simulink model "TGFF_checkout"  (Simulink 9.2)
settings: Solver=FixedStepDiscrete  StartTime=0.0  StopTime=10  FixedStep=SIM_dt  RelTol=1e-3
values from neighbouring files (symbols this model uses):
  SIM_dt = 0.01    [init_secOrdFilt_checkout.m]    (also in init_secOrdSS_checkout.m = 0.001)
undefined symbols (not defined in the file or in its folder): TGFF_B, TGFF_CmdLim_lb, TGFF_CmdLim_ub, TGFF_Coul_Nm, TGFF_Gain, TGFF_J, TGFF_K, TGFF_Kf, TGFF_MomArm, TGFF_Visc_Nmsprad
libraries: simulink x1
settings Model: Creator=coewal  LastModifiedBy=coewal
settings DataIOCC: LimitDataPoints=off  SaveFormat=Dataset  SignalLoggingSaveFormat=Dataset
settings OptimizationCC: LifeSpan=auto
settings DebuggingCC: UnderspecifiedInitializationDetection=Simplified  MergeDetectMultiDrivingBlocksExec=error  FcnCallInpInsideContextMsg=error  StateNameClashWarn=none  SFUnexpectedBacktrackingDiag=error  SFNoUnconditionalDefaultTransitionDiag=error  SFExecutionAtInitializationDiag=warning
settings HardwareCC: ProdBitPerPointer=64  ProdBitPerSizeT=64  ProdBitPerPtrDiffT=64  ProdLargestAtomicFloat=Float  ProdIntDivRoundTo=Zero  ProdEndianess=LittleEndian  ProdWordSize=64  ProdHWDeviceType=Intel->x86-64 (Windows64)
settings ModelReferenceCC: PropagateSignalLabelsOutOfModel=on
settings SFSimCC: SimUseLocalCustomCode=on
settings RTWCC: RTWUseLocalCustomCode=on
settings CodeAppCC: StateflowObjectComments=off
settings GRTTargetCC: TargetLangStandard=C99 (ISO)  GeneratePreprocessorConditionals=Use local settings  CombineOutputUpdateFcns=on  GRTInterface=off
settings ConfigComp: CovMetricSettings=dwe  CovHtmlReporting=off  CovSaveCumulativeToWorkspaceVar=off  CovSaveSingleToWorkspaceVar=off  CovExternalEMLEnable=on

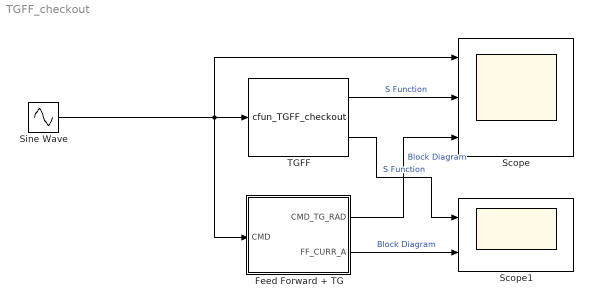
== system TGFF_checkout ==
  Feed Forward + TG : Subsystem
  Scope : Scope  NumInputPorts=3
  Scope1 : Scope  NumInputPorts=2
  Sine Wave : Sin  Amplitude=pi/180  Frequency=5  SampleTime=SIM_dt
  TGFF : S-Function  FunctionName=cfun_TGFF_checkout  Parameters=SIM_dt,TGFF_K,TGFF_B,TGFF_J,TGFF_MomArm,TGFF_Kf,TGFF_Gain,TGFF_CmdLim_ub,TGFF_CmdLim_lb,TGFF_Coul_Nm,TGFF_Visc_Nmsprad  SFunctionModules='TGFF'  SFunctionDeploymentMode=off  EnableBusSupport=off
  wires:
  TGFF/1 -> Scope/2  "S Function"
  Sine Wave/1 -> Feed Forward + TG/1(CMD), Scope/1, TGFF/1
  Feed Forward + TG/2(FF_CURR_A) -> Scope1/2  "Block Diagram"
  Feed Forward + TG/1(CMD_TG_RAD) -> Scope/3  "Block Diagram"
  TGFF/2 -> Scope1/1  "S Function"

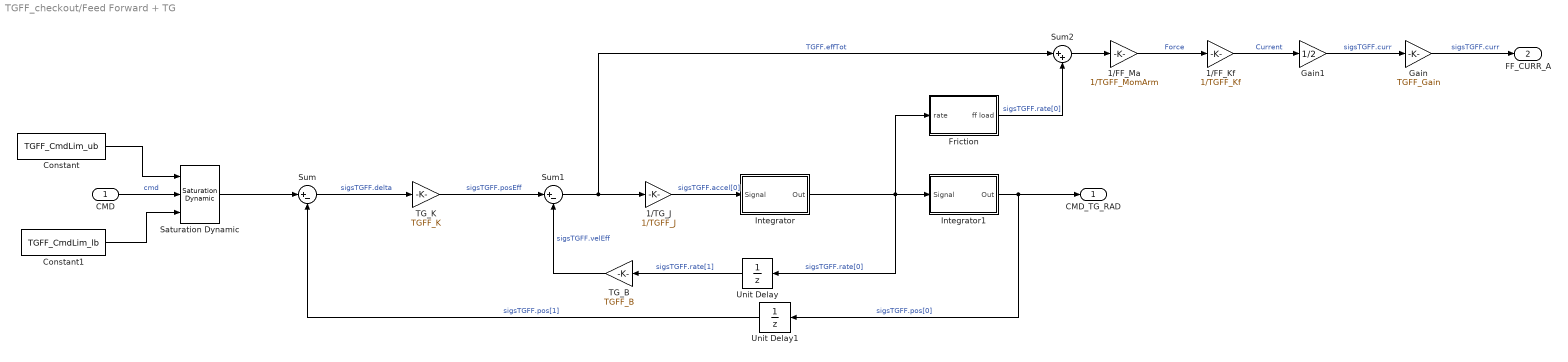
== system TGFF_checkout/Feed Forward + TG ==
  CMD : Inport
  1/FF_Kf : Gain  Gain=1/TGFF_Kf
  1/FF_Ma : Gain  Gain=1/TGFF_MomArm
  1/TG_J : Gain  Gain=1/TGFF_J
  Constant : Constant  Value=TGFF_CmdLim_ub  SampleTime=SIM_dt
  Constant1 : Constant  Value=TGFF_CmdLim_lb  SampleTime=SIM_dt
  Friction : Subsystem
  Gain : Gain  Gain=TGFF_Gain
  Gain1 : Gain  Gain=1/2
  Integrator : Subsystem
  Integrator1 : Subsystem
  Saturation Dynamic : simulink/Discontinuities/Saturation Dynamic  OutMin=[]  OutMax=[]  OutDataTypeStr=Inherit: Same as second input  OutDataType=fixdt(1, 16)  OutScaling=2^-10  DoSatur=off
  Sum : Sum  Inputs=|+-
  Sum1 : Sum  Inputs=|+-
  Sum2 : Sum  Inputs=|++
  TG_B : Gain  Gain=TGFF_B
  TG_K : Gain  Gain=TGFF_K
  Unit Delay : UnitDelay  SampleTime=-1
  Unit Delay1 : UnitDelay  SampleTime=-1
  CMD_TG_RAD : Outport
  FF_CURR_A : Outport  Port=2
  wires:
  CMD/1 -> Saturation Dynamic/2  "cmd"
  Sum/1 -> TG_K/1  "sigsTGFF.delta"
  TG_K/1 -> Sum1/1  "sigsTGFF.posEff"
  Sum1/1 -> Sum2/1, 1/TG_J/1  "TGFF.effTot"
  1/TG_J/1 -> Integrator/1(Signal)  "sigsTGFF.accel[0]"
  Integrator/1(Out) -> Friction/1(rate), Integrator1/1(Signal), Unit Delay/1  "sigsTGFF.rate[0]"
  Integrator1/1(Out) -> Unit Delay1/1, CMD_TG_RAD/1  "sigsTGFF.pos[0]"
  1/FF_Kf/1 -> Gain1/1  "Current"
  Gain/1 -> FF_CURR_A/1  "sigsTGFF.curr"
  Gain1/1 -> Gain/1  "sigsTGFF.curr"
  TG_B/1 -> Sum1/2  "sigsTGFF.velEff"
  Unit Delay/1 -> TG_B/1  "sigsTGFF.rate[1]"
  Unit Delay1/1 -> Sum/2  "sigsTGFF.pos[1]"
  Saturation Dynamic/1 -> Sum/1
  Constant/1 -> Saturation Dynamic/1
  Constant1/1 -> Saturation Dynamic/3
  Friction/1(ff load) -> Sum2/2  "sigsTGFF.rate[0]"
  Sum2/1 -> 1/FF_Ma/1
  1/FF_Ma/1 -> 1/FF_Kf/1  "Force"

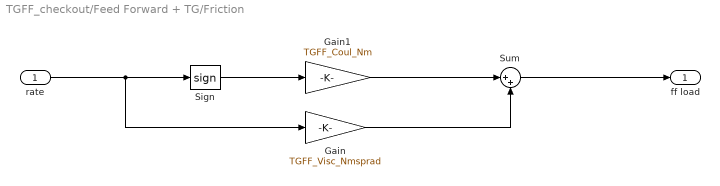
== system TGFF_checkout/Feed Forward + TG/Friction ==
  rate : Inport
  Gain : Gain  DisableCoverage=on  Gain=TGFF_Visc_Nmsprad  SaturateOnIntegerOverflow=on  OutDataTypeStr=Inherit: Same as input
  Gain1 : Gain  DisableCoverage=on  Gain=TGFF_Coul_Nm  OutDataTypeStr=Inherit: Inherit via back propagation  SaturateOnIntegerOverflow=on
  Sign : Signum  DisableCoverage=on
  Sum : Sum  Inputs=|++  SaturateOnIntegerOverflow=on  InputSameDT=on  OutDataTypeStr=Inherit: Same as first input
  ff load : Outport
  wires:
  Sign/1 -> Gain1/1
  rate/1 -> Sign/1, Gain/1
  Gain1/1 -> Sum/1
  Gain/1 -> Sum/2
  Sum/1 -> ff load/1

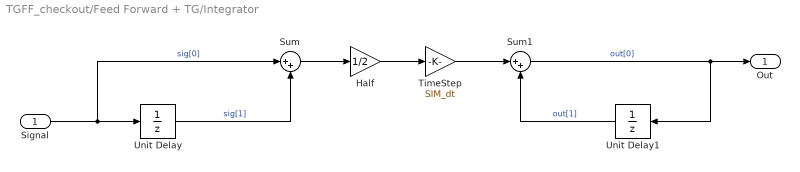
== system TGFF_checkout/Feed Forward + TG/Integrator ==
  Signal : Inport
  Half : Gain  Gain=1/2
  Sum : Sum  Inputs=|++
  Sum1 : Sum  Inputs=|++
  TimeStep : Gain  Gain=SIM_dt
  Unit Delay : UnitDelay  SampleTime=-1
  Unit Delay1 : UnitDelay  SampleTime=-1
  Out : Outport
  wires:
  Signal/1 -> Sum/1, Unit Delay/1  "sig[0]"
  Unit Delay/1 -> Sum/2  "sig[1]"
  Sum/1 -> Half/1
  Half/1 -> TimeStep/1
  TimeStep/1 -> Sum1/1
  Sum1/1 -> Unit Delay1/1, Out/1  "out[0]"
  Unit Delay1/1 -> Sum1/2  "out[1]"

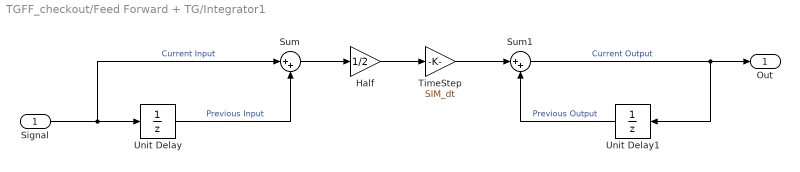
== system TGFF_checkout/Feed Forward + TG/Integrator1 ==
  Signal : Inport
  Half : Gain  Gain=1/2
  Sum : Sum  Inputs=|++
  Sum1 : Sum  Inputs=|++
  TimeStep : Gain  Gain=SIM_dt
  Unit Delay : UnitDelay  SampleTime=-1
  Unit Delay1 : UnitDelay  SampleTime=-1
  Out : Outport
  wires:
  Unit Delay1/1 -> Sum1/2  "Previous Output"
  Sum1/1 -> Out/1, Unit Delay1/1  "Current Output"
  TimeStep/1 -> Sum1/1
  Half/1 -> TimeStep/1
  Sum/1 -> Half/1
  Unit Delay/1 -> Sum/2  "Previous Input"
  Signal/1 -> Unit Delay/1, Sum/1  "Current Input"
